simulink model "Plant"  (R2024b)
settings: Solver=FixedStepAuto  StartTime=0  StopTime=Tend  FixedStep=Tsim  RelTol=1e-3
values from neighbouring files (symbols this model uses):
  alpha_s = wrapToPi(2*pi/m*ps)    [setup.m]    (also in setup_actuator_2026.m; setup_ismb_19.m)
  alpha_t = wrapToPi(2*pi/m*p)    [setup.m]    (also in setup_actuator_2026.m; setup_ismb_19.m)
  Fx_hat = 2*Fx_hat    (= 1.2)    [setup.m]    (also in setup_actuator_2026.m = 2.18026; setup_ismb_19.m)
  Fy_hat = 2*Fy_hat    (= 1.2)    [setup.m]    (also in setup_actuator_2026.m = 2.18026; setup_ismb_19.m)
  lambda_pm = 0.00667    [setup.m]
  p = 4    [setup.m]    (also in setup_actuator_2026.m = 7; setup_ismb_19.m)
  tau_hat = 2*tau_hat    (= 0.0133333333333)    [setup.m]    (also in setup_actuator_2026.m = 0.0649102; setup_ismb_19.m)
  Tsim = 1e-5    (= 1e-05)    [setup.m]    (also in setup_actuator_2026.m = 2e-05; setup_ismb_19.m)
  winding_conf_num = winding_conf_dic(winding_configuration)    [setup.m]    (also in setup_actuator_2026.m; setup_ismb_19.m)
libraries: spsControlledVoltageSourceLib x12, spsCurrentMeasurementLib x6, spsMutualInductanceLib x1, spspowerguiLib x1
settings Model: Creator=chiba  LastModifiedBy=tnoguchi
settings SolverCC: AllowMultiTaskInputOutput=on
settings DataIOCC: SaveOutput=off  SaveTime=off
settings OptimizationCC: DefaultParameterBehavior=Inlined  ReuseModelBlockBuffer=off  EnhancedBackFolding=on  PassReuseOutputArgsAs=Individual arguments  ZeroExternalMemoryAtStartup=off  ZeroInternalMemoryAtStartup=off  OptimizeBlockOrder=speed  DifferentSizesBufferReuse=on  EfficientTunableParamExpr=on
settings DebuggingCC: ParameterTunabilityLossMsg=error
settings SFSimCC: MATLABDynamicMemAlloc=off
settings RTWCC: Description=Embedded Coder  SystemTargetFile=ert.tlc  TemplateMakefile=ert_default_tmf  GPUComputeCapability=3.5
settings CodeAppCC: ForceParamTrailComments=on  IgnoreCustomStorageClasses=off  OperatorAnnotations=on  SimulinkDataObjDesc=on  SFDataObjDesc=on  InsertBlockDesc=on
settings ERTTargetCC: TargetLangStandard=C99 (ISO)  ERTCustomFileTemplate=example_file_process.tlc  DynamicArrayContainerType=coder::array

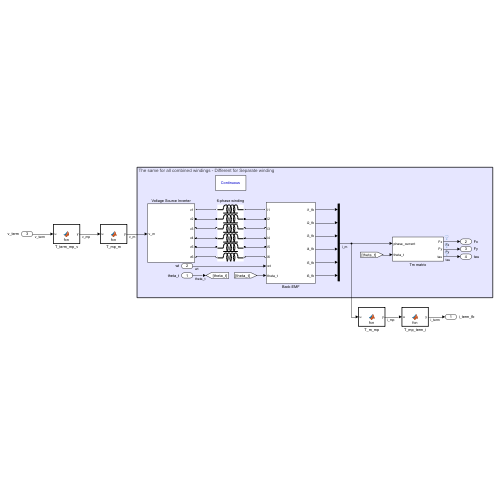
[thumbnail: Simulink's stored preview of the top-level diagram]
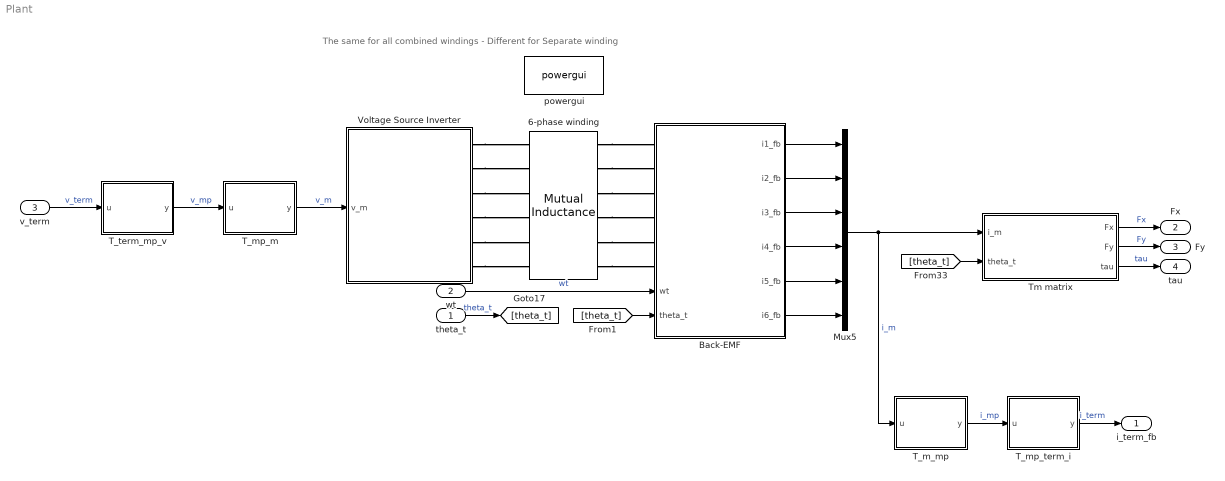
== system Plant ==
  note: The same for all combined windings - Different for Separate winding
  theta_t : Inport  OutDataTypeStr=double  PortDimensions=1  SampleTime=0
  wt : Inport  Port=2  OutDataTypeStr=double  PortDimensions=1
  v_term : Inport  Port=3  OutDataTypeStr=double  PortDimensions=[6 1]  SampleTime=0
  6-phase winding : spsMutualInductanceLib/Mutual Inductance  LConnTagsString=a|b|c|L4|L5|L6  RConnTagsString=A|B|C|R4|R5|R6  TypeOfMutual=Generalized mutual inductance  NumberOfWindings=6  SelfImpedance1=[1.1 1.1e-03]  SelfImpedance2=[ 1.1 1.1e-03]  ThreeWindings=on  SelfImpedance3=[ 1.1 1.1e-03]  MutualImpedance=[1.0 1.0e-03]  InductanceMatrix=Lmat  ResistanceMatrix=Rmat  Measurements=None
      settings: LibrarySourceBlock=sps_lib/Passives/Mutual Inductance
  Back-EMF : Subsystem
      settings: PortSchema="{\"entries\":[{\"content\":{\"sides\":[{\"content\":{\"connectorIds\":[\"LConn1\",\"LConn2\",\"LConn3\",\"LConn4\",\"LConn5\",\"LConn6\",\"In1\",\"In2\"]},\"type\":\"ConnectorPlacement.EquallySpacedRectSide\",\"uuid\":\"749577e6-e43c-48b0-9a92-cb274024c2f1\"},{\"content\":{\"connectorIds\":[\"Out1\",\"Out2\",\"Out3\",\"Out4\",\"Out5\",\"Out6\"],\"side\":\"RIGHT\"},\"type\":\"ConnectorPlacement.EquallySpacedRectSide\",\"uuid\":\"b47f9487-f754-4b9c-a86a-8672228b8979\"},{\"content\":{\"side\":\"TOP\"},\"type\":\"ConnectorPlacement.EquallySpacedRectSide\",\"uuid\":\"ca9d39d3-2f68-4271-a0d3-29a08329b066\"}]},\"type\":\"ConnectorPlacement.EquallySpacedConnector\",\"uuid\":\"24c892f7-b8cb-4be8-a5cc-492343e32fdb\"}],\"packageUris\":[\"http://schema.mathworks.com/mf0/Connector/R2020b\"],\"version\":\"1.0\"}"
  Mux5 : Mux  Inputs=6
  T_m_mp : MATLAB Function  TreatAsAtomicUnit=on
  T_mp_m : MATLAB Function  TreatAsAtomicUnit=on
  T_mp_term_i : MATLAB Function  TreatAsAtomicUnit=on
  T_term_mp_v : MATLAB Function  TreatAsAtomicUnit=on
  Tm matrix : Subsystem
  Voltage Source Inverter : Subsystem
  powergui : spspowerguiLib/powergui  Priority=1  SimulationMode=Continuous  SampleTime=Tsim  frequency=60  Iterations=50  frequencyindice=0  Pbase=100e6  ErrMax=1e-4  UnitsV=kV  UnitsW=MW  buscounter=0  FunctionMessages=off  echomessages=off  EnableUseOfTLC=off  CurrentSourceSwitches=off  DisableSnubberDevices=off  DisableRonSwitches=off  DisableVfSwitches=off  DisplayEquations=off  AutomaticDiscreteSolvers=off  SolverType=Tustin/Backward Euler (TBE)  Interpol=off  ExternalGateDelay=off  methode=off  Ts=100  x0status=blocks  SPID=on  SwTol=0  HookPort=off  NonlinearTolerance=1e-4  nMaxIteration=100  ContinueOnMaxIteration=off  RestoreLinks=warning  ResistiveCurrentMeasurement=off  Frange=[0:2:500]  Ylog=off  Xlog=on  ShowGrid=off  save=off  variable=ZData  structure=0  ZoomFFT=off  StartTime=0.0  cycles=1  DisplayStyle=1  fundamental=60  FreqAxis=off  MaxFrequency=1000  frequencyindicesteady=1  RmsSteady=1  display=off
  i_term_fb : Outport  OutDataTypeStr=double  PortDimensions=6  SampleTime=0
  Fx : Outport  Port=2  OutDataTypeStr=double  PortDimensions=1  SampleTime=0
  Fy : Outport  Port=3  OutDataTypeStr=double  PortDimensions=1  SampleTime=0
  tau : Outport  Port=4  OutDataTypeStr=double  PortDimensions=1  SampleTime=0
  wires:
  Back-EMF/1(i1_fb) -> Mux5/1
  Back-EMF/3(i3_fb) -> Mux5/3
  Back-EMF/2(i2_fb) -> Mux5/2
  Back-EMF/5(i5_fb) -> Mux5/5
  Back-EMF/4(i4_fb) -> Mux5/4
  Back-EMF/6(i6_fb) -> Mux5/6
  [theta_t] -> Tm matrix/2(theta_t)
  Mux5/1 -> Tm matrix/1(i_m), T_m_mp/1(u)  "i_m"
  wt/1 -> Back-EMF/1(wt)  "wt"
  [theta_t] -> Back-EMF/2(theta_t)
  theta_t/1 -> [theta_t]  "theta_t"
  Tm matrix/1(Fx) -> Fx/1  "Fx"
  Tm matrix/2(Fy) -> Fy/1  "Fy"
  Tm matrix/3(tau) -> tau/1  "tau"
  T_term_mp_v/1(y) -> T_mp_m/1(u)  "v_mp"
  v_term/1 -> T_term_mp_v/1(u)  "v_term"
  T_mp_m/1(y) -> Voltage Source Inverter/1(v_m)  "v_m"
  T_m_mp/1(y) -> T_mp_term_i/1(u)  "i_mp"
  T_mp_term_i/1(y) -> i_term_fb/1  "i_term"
  connections:
  6-phase winding/RConn1 -- Back-EMF/LConn1
  6-phase winding/RConn2 -- Back-EMF/LConn2
  6-phase winding/RConn3 -- Back-EMF/LConn3
  6-phase winding/RConn4 -- Back-EMF/LConn4
  6-phase winding/RConn5 -- Back-EMF/LConn5
  6-phase winding/RConn6 -- Back-EMF/LConn6
  Voltage Source Inverter/RConn1 -- 6-phase winding/LConn1
  Voltage Source Inverter/RConn2 -- 6-phase winding/LConn2
  Voltage Source Inverter/RConn3 -- 6-phase winding/LConn3
  Voltage Source Inverter/RConn4 -- 6-phase winding/LConn4
  Voltage Source Inverter/RConn5 -- 6-phase winding/LConn5
  Voltage Source Inverter/RConn6 -- 6-phase winding/LConn6

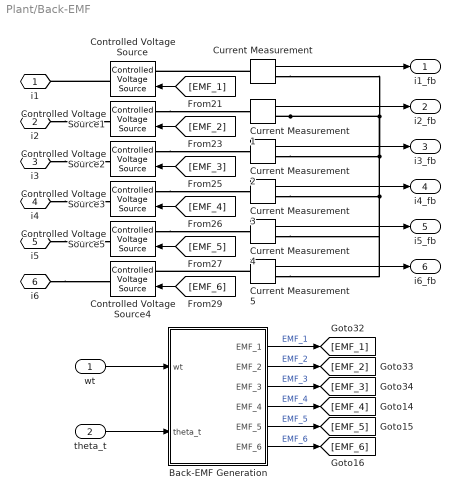
== system Plant/Back-EMF ==
  wt : Inport
  theta_t : Inport  Port=2
  Back-EMF Generation : MATLAB Function  TreatAsAtomicUnit=on
  Controlled Voltage Source{,1..5} (6 alike) : spsControlledVoltageSourceLib/Controlled Voltage Source  Initialize=on  Source_Type=AC  Amplitude=0  Phase=0  Frequency=0  Measurements=None
  Current Measurement{,1..5} (6 alike) : spsCurrentMeasurementLib/Current Measurement  PhasorSimulation=off  OutputType=Complex  PSBequivalent=0
  i1 : PMIOPort  Side=Left
  i2 : PMIOPort  Port=2  Side=Left
  i3 : PMIOPort  Port=3  Side=Left
  i4 : PMIOPort  Port=4  Side=Left
  i5 : PMIOPort  Port=5  Side=Left
  i6 : PMIOPort  Port=6  Side=Left
  i1_fb : Outport
  i2_fb : Outport  Port=2
  i3_fb : Outport  Port=3
  i4_fb : Outport  Port=4
  i5_fb : Outport  Port=5
  i6_fb : Outport  Port=6
  wires:
  Current Measurement2/1 -> i3_fb/1
  Current Measurement4/1 -> i5_fb/1
  Back-EMF Generation/6(EMF_6) -> [EMF_6]  "EMF_6"
  [EMF_4] -> Controlled Voltage Source3/1
  Current Measurement1/1 -> i2_fb/1
  Back-EMF Generation/5(EMF_5) -> [EMF_5]  "EMF_5"
  Current Measurement3/1 -> i4_fb/1
  Back-EMF Generation/2(EMF_2) -> [EMF_2]  "EMF_2"
  [EMF_2] -> Controlled Voltage Source1/1
  [EMF_3] -> Controlled Voltage Source2/1
  [EMF_1] -> Controlled Voltage Source/1
  Current Measurement/1 -> i1_fb/1
  Back-EMF Generation/3(EMF_3) -> [EMF_3]  "EMF_3"
  Back-EMF Generation/4(EMF_4) -> [EMF_4]  "EMF_4"
  [EMF_6] -> Controlled Voltage Source4/1
  Back-EMF Generation/1(EMF_1) -> [EMF_1]  "EMF_1"
  wt/1 -> Back-EMF Generation/1(wt)
  [EMF_5] -> Controlled Voltage Source5/1
  theta_t/1 -> Back-EMF Generation/2(theta_t)
  Current Measurement5/1 -> i6_fb/1
  connections:
  i5/RConn1 -- Controlled Voltage Source5/RConn1
  i3/RConn1 -- Controlled Voltage Source2/RConn1
  Controlled Voltage Source2/LConn1 -- Current Measurement2/LConn1
  i6/RConn1 -- Controlled Voltage Source4/RConn1
  i4/RConn1 -- Controlled Voltage Source3/RConn1
  Controlled Voltage Source1/LConn1 -- Current Measurement1/LConn1
  Current Measurement1/RConn1 -- Current Measurement3/RConn1 -- Current Measurement5/RConn1 -- Current Measurement4/RConn1 -- Current Measurement2/RConn1 -- Current Measurement/RConn1
  Controlled Voltage Source/RConn1 -- i1/RConn1
  Current Measurement/LConn1 -- Controlled Voltage Source/LConn1
  Controlled Voltage Source3/LConn1 -- Current Measurement3/LConn1
  i2/RConn1 -- Controlled Voltage Source1/RConn1
  Controlled Voltage Source5/LConn1 -- Current Measurement4/LConn1
  Current Measurement5/LConn1 -- Controlled Voltage Source4/LConn1

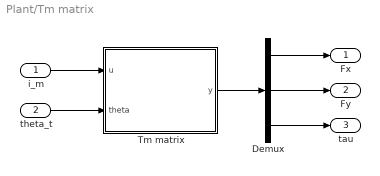
== system Plant/Tm matrix ==
  i_m : Inport
  theta_t : Inport  Port=2
  Demux : Demux  Outputs=3
  Tm matrix : MATLAB Function  TreatAsAtomicUnit=on
  Fx : Outport
  Fy : Outport  Port=2
  tau : Outport  Port=3
  wires:
  i_m/1 -> Tm matrix/1(u)
  Tm matrix/1(y) -> Demux/1
  Demux/1 -> Fx/1
  Demux/2 -> Fy/1
  Demux/3 -> tau/1
  theta_t/1 -> Tm matrix/2(theta)

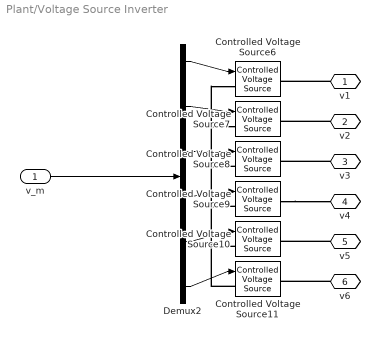
== system Plant/Voltage Source Inverter ==
  v_m : Inport
  Controlled Voltage Source{6..11} (6 alike) : spsControlledVoltageSourceLib/Controlled Voltage Source  Initialize=on  Source_Type=AC  Amplitude=0  Phase=0  Frequency=0  Measurements=None
  Demux2 : Demux  Outputs=6
  v1 : PMIOPort  Side=Right
  v2 : PMIOPort  Port=2  Side=Right
  v3 : PMIOPort  Port=3  Side=Right
  v4 : PMIOPort  Port=4  Side=Right
  v5 : PMIOPort  Port=5  Side=Right
  v6 : PMIOPort  Port=6  Side=Right
  wires:
  Demux2/1 -> Controlled Voltage Source6/1
  Demux2/6 -> Controlled Voltage Source11/1
  Demux2/4 -> Controlled Voltage Source9/1
  Demux2/3 -> Controlled Voltage Source8/1
  v_m/1 -> Demux2/1
  Demux2/5 -> Controlled Voltage Source10/1
  Demux2/2 -> Controlled Voltage Source7/1
  connections:
  Controlled Voltage Source11/LConn1 -- Controlled Voltage Source10/LConn1 -- Controlled Voltage Source9/LConn1 -- Controlled Voltage Source6/LConn1 -- Controlled Voltage Source7/LConn1 -- Controlled Voltage Source8/LConn1
  v2/RConn1 -- Controlled Voltage Source7/RConn1
  v6/RConn1 -- Controlled Voltage Source11/RConn1
  v1/RConn1 -- Controlled Voltage Source6/RConn1
  Controlled Voltage Source9/RConn1 -- v4/RConn1
  v3/RConn1 -- Controlled Voltage Source8/RConn1
  v5/RConn1 -- Controlled Voltage Source10/RConn1

== matlab function Plant/T_m_mp ==
  data: u input; y output; T_m_mp parameter
function y  = fcn(u, T_m_mp)

y = T_m_mp*u;

== matlab function Plant/Back-EMF/Back-EMF Generation ==
  data: EMF_1 output; EMF_2 output; EMF_3 output; EMF_4 output; EMF_5 output; EMF_6 output; wt input; theta_t input; lambda_pm parameter; p parameter; alpha_t parameter; winding_conf_num parameter
function [EMF_1, EMF_2, EMF_3, EMF_4, EMF_5, EMF_6] = fcn(wt, theta_t, lambda_pm, p, alpha_t, winding_conf_num)

if winding_conf_num == 1
    alpha = 2*pi/3;
    EMF_1 = (wt/p)*lambda_pm*sin(0-theta_t);
    EMF_2 = (wt/p)*lambda_pm*sin(alpha-theta_t);
    EMF_3 = (wt/p)*lambda_pm*sin(2*alpha-theta_t);
    EMF_4 = 0;
    EMF_5 = 0;
    EMF_6 = 0;
else
    EMF_1 = (wt/p)*lambda_pm*sin(0-theta_t);
    EMF_2 = (wt/p)*lambda_pm*sin(alpha_t-theta_t);
    EMF_3 = (wt/p)*lambda_pm*sin(2*alpha_t-theta_t);
    EMF_4 = (wt/p)*lambda_pm*sin(3*alpha_t-theta_t);
    EMF_5 = (wt/p)*lambda_pm*sin(4*alpha_t-theta_t);
    EMF_6 = (wt/p)*lambda_pm*sin(5*alpha_t-theta_t);
end

end

== matlab function Plant/T_mp_term_i ==
  data: u input; y output; T_mp_term_i parameter
function y  = fcn(u, T_mp_term_i)

y = T_mp_term_i*u;

== matlab function Plant/T_mp_m ==
  data: u input; y output; T_mp_m parameter
function y  = fcn(u, T_mp_m)

y = T_mp_m*u;

== matlab function Plant/T_term_mp_v ==
  data: u input; y output; T_term_mp_v parameter
function y  = fcn(u, T_term_mp_v)

y = T_term_mp_v*u;

== matlab function Plant/Tm matrix/Tm matrix ==
  data: u input; y output; theta input; alpha_t parameter; alpha_s parameter; tau_hat parameter; Fx_hat parameter; Fy_hat parameter; winding_conf_num parameter
function y = fcn(u, theta, alpha_t, alpha_s, tau_hat, Fx_hat, Fy_hat, winding_conf_num)

if winding_conf_num == 1
    alpha = 2*pi/3;
    Tm = [0 0 0 Fx_hat*cos(theta) Fx_hat*cos(theta-alpha) Fx_hat*cos(theta-2*alpha);
          0 0 0 Fy_hat*sin(theta) Fy_hat*sin(theta-alpha) Fy_hat*sin(theta-2*alpha);
          -tau_hat*sin(theta) -tau_hat*sin(theta-alpha) -tau_hat*sin(theta-2*alpha) 0 0 0];
else
    Tm = [Fx_hat*cos(theta) Fx_hat*cos(theta-alpha_s) Fx_hat*cos(theta-2*alpha_s) Fx_hat*cos(theta-3*alpha_s) Fx_hat*cos(theta-4*alpha_s) Fx_hat*cos(theta-5*alpha_s);
          Fy_hat*sin(theta) Fy_hat*sin(theta-alpha_s) Fy_hat*sin(theta-2*alpha_s) Fy_hat*sin(theta-3*alpha_s) Fy_hat*sin(theta-4*alpha_s) Fy_hat*sin(theta-5*alpha_s);
          -tau_hat*sin(theta) -tau_hat*sin(theta-alpha_t) -tau_hat*sin(theta-2*alpha_t) -tau_hat*sin(theta-3*alpha_t) -tau_hat*sin(theta-4*alpha_t) -tau_hat*sin(theta-5*alpha_t)];
end

y = Tm*u;

end
